simulink model "clarke_park_transformations"  (R2020b)
settings: Solver=VariableStepAuto  StartTime=0.0  StopTime=10.0  RelTol=1e-3
undefined symbols (not defined in the file or in its folder): f_rad, V_g
libraries: simulink x3
settings Model: Creator=martin  LastModifiedBy=martin

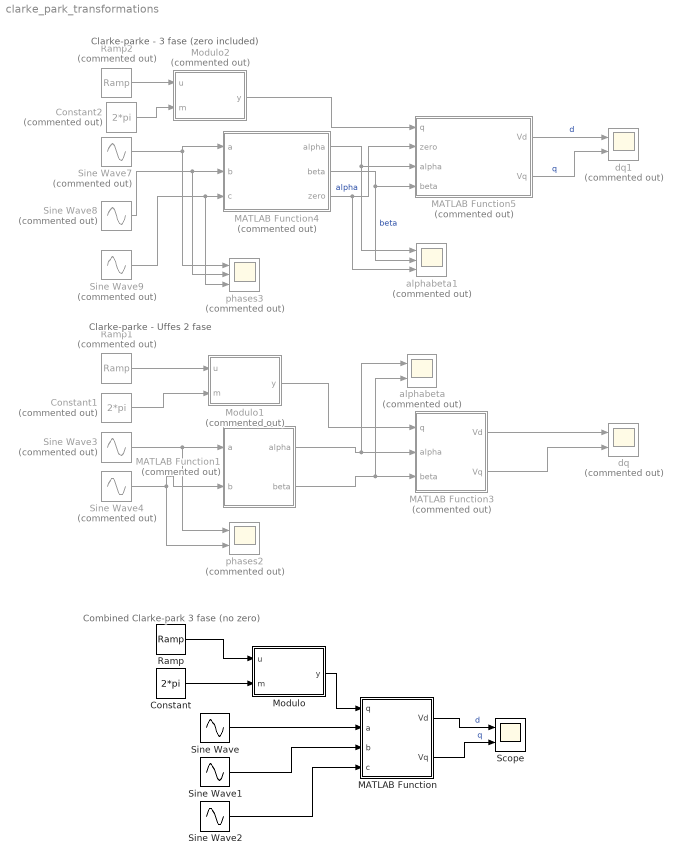
== system clarke_park_transformations ==
  note: Clarke-parke - Uffes 2 fase
  note: Combined Clarke-park 3 fase (no zero)
  note: Clarke-parke - 3 fase (zero included)
  Constant : Constant  Value=2*pi
  Constant1 : Constant  Commented=on  Value=2*pi
  Constant2 : Constant  Commented=on  Value=2*pi
  MATLAB Function : MATLAB Function  TreatAsAtomicUnit=on
  MATLAB Function1 : MATLAB Function  Commented=on  TreatAsAtomicUnit=on
  MATLAB Function3 : MATLAB Function  Commented=on  TreatAsAtomicUnit=on
  MATLAB Function4 : MATLAB Function  Commented=on  TreatAsAtomicUnit=on
  MATLAB Function5 : MATLAB Function  Commented=on  TreatAsAtomicUnit=on
  Modulo : MATLAB Function  TreatAsAtomicUnit=on
  Modulo1 : MATLAB Function  Commented=on  TreatAsAtomicUnit=on
  Modulo2 : MATLAB Function  Commented=on  TreatAsAtomicUnit=on
  Ramp : simulink/Sources/Ramp  slope=f_rad  start=0  InitialOutput=-pi/2
  Ramp1 : simulink/Sources/Ramp  Commented=on  slope=50*2*pi  start=0  InitialOutput=0
  Ramp2 : simulink/Sources/Ramp  Commented=on  slope=50*2*pi  start=0  InitialOutput=0
  Scope : Scope  NumInputPorts=2
  Sine Wave : Sin  Amplitude=V_g  Frequency=f_rad  SampleTime=0
  Sine Wave1 : Sin  Amplitude=V_g  Frequency=f_rad  Phase=-120*pi/180  SampleTime=0
  Sine Wave2 : Sin  Amplitude=V_g  Frequency=f_rad  Phase=120*pi/180  SampleTime=0
  Sine Wave3 : Sin  Commented=on  Amplitude=230  Frequency=50*2*pi  SampleTime=0
  Sine Wave4 : Sin  Commented=on  Amplitude=230  Frequency=50*2*pi  Phase=-120*pi/180  SampleTime=0
  Sine Wave7 : Sin  Commented=on  Amplitude=230  Frequency=50*2*pi  SampleTime=0
  Sine Wave8 : Sin  Commented=on  Amplitude=230  Frequency=50*2*pi  Phase=-120*pi/180  SampleTime=0
  Sine Wave9 : Sin  Commented=on  Amplitude=230  Frequency=50*2*pi  Phase=120*pi/180  SampleTime=0
  alphabeta : Scope  Commented=on  NumInputPorts=2
  alphabeta1 : Scope  Commented=on  NumInputPorts=3
  dq : Scope  Commented=on  NumInputPorts=2
  dq1 : Scope  Commented=on  NumInputPorts=2
  phases2 : Scope  Commented=on  NumInputPorts=2
  phases3 : Scope  Commented=on  NumInputPorts=3
  wires:
  MATLAB Function5/2(Vq) -> dq1/2  "q"
  Constant1/1 -> Modulo1/2(m)
  Sine Wave2/1 -> MATLAB Function/4(c)
  MATLAB Function1/1(alpha) -> alphabeta/1, MATLAB Function3/2(alpha)
  MATLAB Function3/1(Vd) -> dq/1
  Modulo1/1(y) -> MATLAB Function3/1(q)
  MATLAB Function4/3(zero) -> alphabeta1/3, MATLAB Function5/2(zero)
  Modulo/1(y) -> MATLAB Function/1(q)
  Sine Wave9/1 -> phases3/3, MATLAB Function4/3(c)
  Constant2/1 -> Modulo2/2(m)
  MATLAB Function4/2(beta) -> alphabeta1/2, MATLAB Function5/4(beta)  "beta"
  Ramp2/1 -> Modulo2/1(u)
  Constant/1 -> Modulo/2(m)
  MATLAB Function/1(Vd) -> Scope/1  "d"
  MATLAB Function1/2(beta) -> alphabeta/2, MATLAB Function3/3(beta)
  Sine Wave8/1 -> phases3/2, MATLAB Function4/2(b)
  Sine Wave7/1 -> MATLAB Function4/1(a), phases3/1
  MATLAB Function5/1(Vd) -> dq1/1  "d"
  MATLAB Function3/2(Vq) -> dq/2
  MATLAB Function/2(Vq) -> Scope/2  "q"
  Sine Wave3/1 -> phases2/1, MATLAB Function1/1(a)
  Sine Wave4/1 -> MATLAB Function1/2(b), phases2/2
  MATLAB Function4/1(alpha) -> alphabeta1/1, MATLAB Function5/3(alpha)  "alpha"
  Ramp1/1 -> Modulo1/1(u)
  Sine Wave/1 -> MATLAB Function/2(a)
  Modulo2/1(y) -> MATLAB Function5/1(q)
  Sine Wave1/1 -> MATLAB Function/3(b)
  Ramp/1 -> Modulo/1(u)

== matlab function clarke_park_transformations/MATLAB Function1 ==
  data: alpha output; a input; beta output; b input
function [alpha, beta] = ab_alphabeta(a, b)

Valphabeta = [a; (1/sqrt(3)) * a + (2/sqrt(3)) *b]

alpha = Valphabeta(1,:)
beta = Valphabeta(2,:)

== matlab function clarke_park_transformations/MATLAB Function ==
  data: Vd output; q input; a input; Vq output; b input; c input
function [Vd,Vq] = abc_dq(q, a, b, c)

% 2/3 in stead of sqrt(2/3)!

Vabc = [a;b;c]
Vdq = 2/3*[cos(q) cos(q-2*pi/3) cos(q+2*pi/3); 
     -sin(q) -sin(q-2*pi/3) -sin(q+2*pi/3)] * Vabc

Vd = Vdq(1,:)
Vq = Vdq(2,:)

== matlab function clarke_park_transformations/Modulo ==
  data: u input; y output; m input
function y = modulo(u, m)

y = mod(u,m);

== matlab function clarke_park_transformations/MATLAB Function3 ==
  data: Vd output; q input; Vq output; alpha input; beta input
function [Vd, Vq] = alphabeta_dq(q, alpha, beta)

Vdq = [alpha*cos(q)+beta*sin(q); -alpha*sin(q)+beta*cos(q)]

Vd = Vdq(1,:)
Vq = Vdq(2,:)

== matlab function clarke_park_transformations/MATLAB Function4 ==
  data: alpha output; a input; beta output; b input; c input; zero output
function [alpha, beta, zero] = abc_alphabetazero(a, b, c)

% 2/3 in stead of sqrt(2/3)!
Valphabeta = 2/3*[1         -1/2        -1/2;
                  0         sqrt(3)/2   -sqrt(3)/2;
                  1/sqrt(2) 1/sqrt(2)   1/sqrt(2)]      * [a;b;c]

alpha = Valphabeta(1,:)
beta = Valphabeta(2,:)
zero = Valphabeta(3,:)

== matlab function clarke_park_transformations/MATLAB Function5 ==
  data: Vd output; q input; zero input; Vq output; alpha input; beta input
function [Vd, Vq] = alpbetzer_dq(q, zero, alpha, beta)

Vdq = [cos(q) sin(q) 0;-sin(q) cos(q) 0;0 0 1]*[alpha;beta;zero]
Vd = Vdq(1,:)
Vq = Vdq(2,:)
zero = Vdq(3,:)

== matlab function clarke_park_transformations/Modulo1 ==
  data: u input; y output; m input
function y = modulo(u, m)

y = mod(u,m);

== matlab function clarke_park_transformations/Modulo2 ==
  data: u input; y output; m input
function y = modulo(u, m)

y = mod(u,m);
